simulink library "base_lib"  (R2023a)
settings: Solver=VariableStepAuto  StartTime=0.0  StopTime=10.0  RelTol=1e-3
(part 4 of 4)

== matlab function base_lib/F0021_R1234yf/F0021_dudrho.m ==
  data: T input; du_drho output; rho input
function du_drho = R1234yf_dudrho(T,rho)
%R1234yf_dudrho
%    DU_DRHO = R1234yf_dudrho(T,RHO)

%    This function was generated by the Symbolic Math Toolbox version 9.3.
%    19-Oct-2023 14:13:06

t2 = rho.^2;
t3 = rho.^3;
t4 = 1.0./T;
t7 = rho./4.17e+3;
t12 = rho.*1.863257595362559e-6;
t15 = rho.*1.173162189672722e-7;
t19 = rho.*6.716928615381076e-7;
t20 = rho.*1.53661243666937e-7;
t21 = rho.*1.213417755004629e-7;
t5 = t4.^2;
t6 = t4.^3;
t8 = -t7;
t9 = t4.*5.8856e+4;
t11 = t4.*3.6785e+2;
t13 = t4.*7.94556e+4;
t14 = t2./1.73889e+7;
t16 = t4.*1.044694e+3;
t17 = t7-4.1e+1./2.5e+1;
t27 = t4.*6.54773e+2;
t28 = t4.*1.699467e+3;
t29 = t7-9.1e+1./1.0e+2;
t30 = t7-8.9e+1./1.25e+2;
t31 = t7-3.59e+2./5.0e+2;
t39 = t7-6.77e+2./1.0e+3;
t60 = t12-1.274244604316547e-2;
t68 = t15-3.483165467625899e-4;
t79 = t19-2.011088729016787e-3;
t81 = t20-5.830983213429257e-4;
t82 = t21-3.425587529976019e-4;
t10 = exp(t8);
t18 = -t14;
t22 = t11.^(2.0./5.0);
t23 = t11.^(5.0./2.0);
t24 = t11.^(7.0./2.0);
t25 = t11.^(7.0./5.0);
t32 = t11-6.0./5.0;
t33 = t11.^(1.0./2.0e+1);
t34 = t17.^2;
t35 = t11.^(1.9e+1./2.5e+1);
t36 = t11.^(3.2e+1./2.5e+1);
t37 = t11.^(3.6e+1./2.5e+1);
t38 = t9-2.048e+2;
t40 = t11-3.2e+1./2.5e+1;
t41 = t11-2.3e+1./5.0e+1;
t42 = 1.0./t11.^(3.0./1.0e+2);
t43 = t29.^2;
t44 = t30.^2;
t45 = t31.^2;
t47 = t11-6.7e+1./1.0e+2;
t48 = t11-1.13e+2./1.0e+2;
t49 = t13-2.592e+2;
t50 = t39.^2;
t63 = t16-3.2092;
t69 = t27-8.188e-1;
t72 = t28-3.0954;
t26 = exp(t18);
t46 = t32.^2;
t51 = t40.^2;
t52 = t41.^2;
t54 = t47.^2;
t55 = t48.^2;
t56 = t34.*(8.1e+1./5.0);
t61 = t44.*(5.1e+1./5.0e+1);
t65 = t45.*(1.46e+2./2.5e+1);
t66 = t43.*(1.67e+2./1.25e+2);
t73 = t50.*(2.11e+2./2.0e+2);
t53 = t46.*1.08e+2;
t58 = -t56;
t59 = t51.*8.0e+1;
t64 = -t61;
t67 = -t65;
t70 = -t66;
t71 = t52.*(8.9e+1./1.0e+2);
t75 = t55.*(7.1e+1./5.0e+1);
t76 = -t73;
t78 = t54.*(2.31e+2./1.0e+2);
t57 = -t53;
t62 = -t59;
t74 = -t71;
t77 = -t75;
t80 = -t78;
t83 = t57+t58;
t85 = t62+t67;
t87 = t64+t77;
t89 = t70+t80;
t90 = t74+t76;
t84 = exp(t83);
t86 = exp(t85);
t88 = exp(t87);
t91 = exp(t89);
t92 = exp(t90);
et1 = t3.*1.858131002604336e-12-t26.*t36.*2.023446617579852;
et2 = t2.*t86.*(-1.452200134424495e-7)-t5.*t91.*1.422328005554134e+5;
et3 = t22.*t88.*1.427255066297698-rho.*t42.^2.*1.59640689065627e-4;
et4 = t2.*1.0./t11.^(3.1e+1./5.0e+1).*8.453302832006239e-9+1.0./t11.^(1.7e+1./2.5e+1).*3.630762837322852e-1;
et5 = 1.0./t11.^(7.1e+1./1.0e+3).*(-1.60479554422836)+rho.^7.*t10.*t33.*9.468704878352454e-28;
et6 = t2.^3.*t10.*t33.*(-2.763914953991081e-23)+t2.^2.*t26.*t35.*5.274136083584932e-15;
et7 = rho.*t10.*t42.*2.322094583878085e-4-rho.*t26.*t37.*5.981304050145462e-4;
et8 = rho.*t23.*t84.*4.221246493387974e-7-t2.*t10.*t42.*2.784286071796265e-8;
et9 = t2.*t26.*t35.*(-1.37567137415775e-7)+t2.*t26.*t36.*2.327285357417493e-7;
et10 = t3.*t26.*t37.*3.439725370866163e-11-t2.*t23.*t92.*8.74770499448078e-8;
et11 = t3.*t79.*t86.*4.840667114748315e-8+t6.*t72.*t91.*1.74401118947696e+7;
et12 = t25.*t63.*t88.*(-1.019467904498356)-rho.*t24.*t49.*t84.*1.206070426682278e-7;
et13 = rho.*t5.*t81.*t91.*1.422328005554134e+5-rho.*t22.*t68.*t88.*1.427255066297698;
et14 = t2.*t4.*t38.*t86.*5.341918194480503e-5-t2.*t23.*t60.*t84.*2.110623246693987e-7;
et15 = t2.*t24.*t69.*t92.*2.499344284137366e-8+t3.*t23.*t82.*t92.*2.915901664826927e-8;
et16 = rho.*t25.*t63.*t68.*t88.*1.019467904498356-rho.*t6.*t72.*t81.*t91.*1.74401118947696e+7;
et17 = t3.*t4.*t38.*t79.*t86.*(-1.780639398160168e-5)+t2.*t24.*t49.*t60.*t84.*6.030352133411391e-8;
et18 = t3.*t24.*t69.*t82.*t92.*(-8.331147613791219e-9);
du_drho = et1+et2+et3+et4+et5+et6+et7+et8+et9+et10+et11+et12+et13+et14+et15+et16+et17+et18;
end

== matlab function base_lib/F0021_R1234yf/F0021_dvapsat.m ==
  data: T input; dvap output
function dvap = F0021_dvapsat(T)

% critical Temp & density
Tc   =     367.85; % [K]
% rhoc =     4170.0; % [mol/m3]

T = min(T, Tc);
T = max(T, 0);

% coefficients
x = [ 8.5116; -7.9050; 1.6189; 2.6394; -1.3847 ];

% saturated vapor density
Tr   = T ./ Tc;
th   = 1 ./ (1 - Tr);
A    = [ ones(size(Tr)), log(th).^(-1.5), log(th).^(-2), log(th).^(-3), log(th).^(-4) ];
dvap = exp(A*x);


end

== matlab function base_lib/F0021_R1234yf/F0021_g.m ==
  data: T input; g output; rho input
function g = F0021_g(T,rho)
%R1234yf_g
%    G = R1234yf_g(T,RHO)

%    This function was generated by the Symbolic Math Toolbox version 9.3.
%    16-Oct-2023 15:47:52

t2 = rho.^2;
t3 = rho.^3;
t5 = rho.^7;
t6 = 1.0./T;
t8 = rho./4.17e+3;
t4 = t2.^2;
t7 = t6.^3;
t9 = -t8;
t11 = t6.*3.6785e+2;
t12 = t2./1.73889e+7;
t13 = t8-4.1e+1./2.5e+1;
t18 = t8-9.1e+1./1.0e+2;
t19 = t8-8.9e+1./1.25e+2;
t20 = t8-3.59e+2./5.0e+2;
t30 = t8-6.77e+2./1.0e+3;
t10 = exp(t9);
t14 = -t12;
t15 = t11.^(7.0./2.0);
t16 = t11.^(7.0./5.0);
t21 = t11-6.0./5.0;
t22 = t13.^2;
t23 = t11.^(8.0./2.5e+1);
t24 = t11.^(2.1e+1./2.0e+1);
t25 = t11.^(1.9e+1./5.0e+1);
t26 = t11.^(4.4e+1./2.5e+1);
t28 = t11.^(6.1e+1./2.5e+1);
t29 = t11.^(4.7e+1./5.0e+1);
t31 = t11-3.2e+1./2.5e+1;
t32 = t11-2.3e+1./5.0e+1;
t33 = t18.^2;
t34 = t19.^2;
t35 = t20.^2;
t37 = t11.^(9.7e+1./1.0e+2);
t38 = t11-6.7e+1./1.0e+2;
t39 = t11-1.13e+2./1.0e+2;
t40 = t30.^2;
t43 = t11.^(9.29e+2./1.0e+3);
t17 = exp(t14);
t27 = t25.^6;
t36 = t21.^2;
t41 = t31.^2;
t42 = t32.^2;
t45 = t38.^2;
t46 = t39.^2;
t47 = t22.*(8.1e+1./5.0);
t51 = t34.*(5.1e+1./5.0e+1);
t54 = t35.*(1.46e+2./2.5e+1);
t55 = t33.*(1.67e+2./1.25e+2);
t59 = t40.*(2.11e+2./2.0e+2);
t76 = t2.*t10.*t37.*3.913566700596357e-8;
t77 = t5.*t10.*t24.*1.229509534838242e-27;
t44 = t36.*1.08e+2;
t49 = -t47;
t50 = t41.*8.0e+1;
t53 = -t51;
t56 = -t54;
t57 = -t55;
t58 = t42.*(8.9e+1./1.0e+2);
t61 = t46.*(7.1e+1./5.0e+1);
t62 = -t59;
t64 = t45.*(2.31e+2./1.0e+2);
t48 = -t44;
t52 = -t50;
t60 = -t58;
t63 = -t61;
t65 = -t64;
t66 = t48+t49;
t68 = t52+t56;
t70 = t53+t63;
t72 = t57+t65;
t73 = t60+t62;
t67 = exp(t66);
t69 = exp(t68);
t71 = exp(t70);
t74 = exp(t72);
t75 = exp(t73);
et1 = t23.*1.546958-t43.*2.355237-t76+t77-rho.*t29.*2.315508393285372e-4+t3.*t6.*9.319180196722149e-10;
et2 = t2.*t25.*3.033007263254145e-8-t17.*t27.*1.210006-t7.*t74.*2.377824987227386e+7+t16.*t71.*1.389966;
et3 = t2.^3.*t10.*t24.*(-3.588938332192827e-23)-rho.*t17.*t28.*3.342232613908873e-4+rho.*t10.*t37.*3.263914628297362e-4+rho.*t15.*t67.*1.644384172661871e-7;
et4 = t2.*t17.*t26.*(-1.06569432224005e-7)+t2.*t17.*t27.*1.391699302428561e-7+t4.*t17.*t26.*4.085726420264459e-15+t3.*t17.*t28.*1.922049476337705e-11;
et5 = t2.*t6.*t69.*(-7.283294189396684e-5)-t2.*t15.*t75.*3.407663509480186e-8-rho.*t16.*t71.*(rho.*4.892086330935252e-4-1.45248).*3.333251798561151e-4;
et6 = rho.*t7.*t74.*(rho.*6.407673860911271e-4-2.43152).*5.702218194789895e+3-t2.*t15.*t67.*(rho.*7.769784172661871e-3-5.3136e+1).*1.971683660266032e-11;
et7 = t3.*t6.*t69.*(rho.*2.800959232613909e-3-8.38624).*5.821977769301905e-9+t3.*t15.*t75.*(rho.*5.059952038369305e-4-1.42847).*2.723951646267135e-12;
et8 = t6.*2.95847224925e+3+t76-t77+log(-exp(t6.*-7.18e+2)+1.0).*7.549+log(-exp(t6.*-8.77e+2)+1.0).*1.537+log(-exp(t6.*-1.755e+3)+1.0).*7.455+log(-exp(t6.*-4.465e+3)+1.0).*(2.03e+2./1.0e+2)+log(t8)+log(t11).*(6.18e+2./1.25e+2)+rho.*t23.*3.709731414868106e-4;
et9 = rho.*t43.*(-5.64805035971223e-4)+t4.*t6.*5.587038487243495e-14+t3.*t25.*2.424466237613225e-12-t2.*t29.*2.776388960773827e-8+t8.*(et1+et2+et3+et4+et5+et6+et7);
et10 = rho.*t17.*t27.*(-2.901693045563549e-4)-rho.*t7.*t74.*5.702218194789895e+3+rho.*t16.*t71.*3.333251798561151e-4-t3.*t17.*t26.*8.518739586251397e-12;
et11 = t2.*t17.*t28.*(-4.007473158164116e-8)-t3.*t6.*t69.*5.821977769301905e-9+t2.*t15.*t67.*1.971683660266032e-11-t3.*t15.*t75.*2.723951646267135e-12;
et12 = -1.1837928e+1;
g = T.*(et8+et9+et10+et11+et12).*8.314472;
end

== matlab function base_lib/F0021_R1234yf/F0021_h.m ==
  data: T input; h output; rho input
function h = F0021_h(T,rho)
%R1234yf_h
%    H = R1234yf_h(T,RHO)

%    This function was generated by the Symbolic Math Toolbox version 9.3.
%    16-Oct-2023 15:47:51

t2 = rho.^2;
t3 = rho.^3;
t5 = rho.^7;
t6 = 1.0./T;
t8 = rho./4.17e+3;
t4 = t2.^2;
t7 = t6.^3;
t9 = t6.*7.18e+2;
t10 = t6.*8.77e+2;
t11 = t6.*1.755e+3;
t12 = t6.*4.465e+3;
t13 = -t8;
t23 = t6.*3.6785e+2;
t24 = t2./1.73889e+7;
t25 = t8-4.1e+1./2.5e+1;
t31 = t8-9.1e+1./1.0e+2;
t32 = t8-8.9e+1./1.25e+2;
t33 = t8-3.59e+2./5.0e+2;
t40 = t8-6.77e+2./1.0e+3;
t14 = -t9;
t15 = -t10;
t16 = -t11;
t17 = -t12;
t18 = exp(t13);
t26 = -t24;
t27 = t23.^(5.0./2.0);
t28 = t23.^(7.0./2.0);
t29 = t23.^(7.0./5.0);
t34 = t23-6.0./5.0;
t35 = t25.^2;
t36 = t23.^(2.1e+1./2.0e+1);
t37 = t23.^(4.4e+1./2.5e+1);
t38 = t23.^(5.7e+1./2.5e+1);
t39 = t23.^(6.1e+1./2.5e+1);
t41 = t23-3.2e+1./2.5e+1;
t42 = t23-2.3e+1./5.0e+1;
t43 = t31.^2;
t44 = t32.^2;
t45 = t33.^2;
t47 = t23.^(9.7e+1./1.0e+2);
t48 = t23-6.7e+1./1.0e+2;
t49 = t23-1.13e+2./1.0e+2;
t50 = t40.^2;
t19 = exp(t14);
t20 = exp(t15);
t21 = exp(t16);
t22 = exp(t17);
t30 = exp(t26);
t46 = t34.^2;
t51 = t41.^2;
t52 = t42.^2;
t54 = t48.^2;
t55 = t49.^2;
t56 = t35.*(8.1e+1./5.0);
t60 = t44.*(5.1e+1./5.0e+1);
t63 = t45.*(1.46e+2./2.5e+1);
t64 = t43.*(1.67e+2./1.25e+2);
t68 = t50.*(2.11e+2./2.0e+2);
t53 = t46.*1.08e+2;
t58 = -t56;
t59 = t51.*8.0e+1;
t62 = -t60;
t65 = -t63;
t66 = -t64;
t67 = t52.*(8.9e+1./1.0e+2);
t70 = t55.*(7.1e+1./5.0e+1);
t71 = -t68;
t73 = t54.*(2.31e+2./1.0e+2);
t57 = -t53;
t61 = -t59;
t69 = -t67;
t72 = -t70;
t74 = -t73;
t75 = t57+t58;
t77 = t61+t65;
t79 = t62+t72;
t81 = t66+t74;
t82 = t69+t71;
t76 = exp(t75);
t78 = exp(t77);
t80 = exp(t79);
t83 = exp(t81);
t84 = exp(t82);
et1 = T.*(-1.344026097594128e-2)-t4.*1.518836071019028e-16+(t19.*1.473476145167867e+1)./(t19-1.0)+(t20.*3.66439853201033)./(t20-1.0)+(t21.*3.556755470980019e+1)./(t21-1.0)+(t22.*2.464034253092293e+1)./(t22-1.0)+t3.*t78.*1.582704300476255e-11;
et2 = rho.*1.0./t23.^(1.7e+1./2.5e+1).*(-1.187114052757794e-4)+rho.*1.0./t23.^(7.1e+1./1.0e+3).*5.247038784172661e-4+t2.*1.0./t23.^(3.0./5.0e+1).*2.609805623127397e-8;
et3 = t3.*1.0./t23.^(3.1e+1./5.0e+1).*(-9.212971702930256e-13)+rho.*t6.^2.*t83.*4.650443002411223e+1-rho.*t23.^(2.0./5.0).*t80.*4.666552517985612e-4;
et4 = rho.*t23.^(3.2e+1./2.5e+1).*t30.*6.615860143884892e-4+t5.*t18.*t23.^(1.0./2.0e+1).*1.290985011580154e-27+t3.*t23.^(1.9e+1./2.5e+1).*t30.*1.499298167180246e-11;
et5 = t2.*t23.^(3.6e+1./2.5e+1).*t30.*9.778234505920443e-8-t2.*t18.*1.0./t23.^(3.0./1.0e+2).*3.796159699578467e-8-t2.*t27.*t76.*6.900892810931111e-11;
et6 = t3.*t27.*t84.*9.533830761934972e-12+rho.*t29.*t80.*(t6.*1.044694e+3-3.2092).*3.333251798561151e-4-rho.*t7.*t83.*(t6.*1.699467e+3-3.0954).*5.702218194789895e+3;
et7 = t3.*t6.*t78.*(t6.*5.8856e+4-2.048e+2).*(-5.821977769301905e-9)+t2.*t28.*t76.*(t6.*7.94556e+4-2.592e+2).*1.971683660266032e-11;
et8 = t3.*t28.*t84.*(t6.*6.54773e+2-8.188e-1).*(-2.723951646267135e-12)-8.042605;
et9 = t3.*t6.*9.319180196722149e-10-t30.*t38.*1.210006-t7.*t83.*2.377824987227386e+7+t29.*t80.*1.389966;
et10 = rho.*t23.^(4.7e+1./5.0e+1).*(-2.315508393285372e-4)+t2.*t23.^(1.9e+1./5.0e+1).*3.033007263254145e-8+t23.^(8.0./2.5e+1).*1.546958-t23.^(9.29e+2./1.0e+3).*2.355237;
et11 = t2.^3.*t18.*t36.*(-3.588938332192827e-23)+rho.*t18.*t47.*3.263914628297362e-4-rho.*t30.*t39.*3.342232613908873e-4+rho.*t28.*t76.*1.644384172661871e-7;
et12 = t5.*t18.*t36.*1.229509534838242e-27-t2.*t18.*t47.*3.913566700596357e-8-t2.*t30.*t37.*1.06569432224005e-7+t2.*t30.*t38.*1.391699302428561e-7;
et13 = t4.*t30.*t37.*4.085726420264459e-15+t3.*t30.*t39.*1.922049476337705e-11-t2.*t6.*t78.*7.283294189396684e-5-t2.*t28.*t84.*3.407663509480186e-8;
et14 = rho.*t29.*t80.*(rho.*4.892086330935252e-4-1.45248).*(-3.333251798561151e-4)+rho.*t7.*t83.*(rho.*6.407673860911271e-4-2.43152).*5.702218194789895e+3;
et15 = t2.*t28.*t76.*(rho.*7.769784172661871e-3-5.3136e+1).*(-1.971683660266032e-11)+t3.*t6.*t78.*(rho.*2.800959232613909e-3-8.38624).*5.821977769301905e-9;
et16 = t3.*t28.*t84.*(rho.*5.059952038369305e-4-1.42847).*2.723951646267135e-12;
h = T.*(t6.*(et1+et2+et3+et4+et5+et6+et7+et8).*(-3.6785e+2)+t8.*(et9+et10+et11+et12+et13+et14+et15+et16)+1.0).*8.314472;
end

== matlab function base_lib/F0021_R1234yf/F0021_p.m ==
  data: T input; p output; rho input
function p = F0021_p(T,rho)
%R1234yf_p
%    P = R1234yf_p(T,RHO)

%    This function was generated by the Symbolic Math Toolbox version 9.3.
%    16-Oct-2023 15:47:49

t2 = rho.^2;
t3 = rho.^3;
t4 = 1.0./T;
t6 = rho./4.17e+3;
t5 = t4.^3;
t7 = -t6;
t9 = t4.*3.6785e+2;
t10 = t2./1.73889e+7;
t11 = t6-4.1e+1./2.5e+1;
t16 = t6-9.1e+1./1.0e+2;
t17 = t6-8.9e+1./1.25e+2;
t18 = t6-3.59e+2./5.0e+2;
t25 = t6-6.77e+2./1.0e+3;
t8 = exp(t7);
t12 = -t10;
t13 = t9.^(7.0./2.0);
t14 = t9.^(7.0./5.0);
t19 = t9-6.0./5.0;
t20 = t11.^2;
t21 = t9.^(2.1e+1./2.0e+1);
t22 = t9.^(4.4e+1./2.5e+1);
t23 = t9.^(5.7e+1./2.5e+1);
t24 = t9.^(6.1e+1./2.5e+1);
t26 = t9-3.2e+1./2.5e+1;
t27 = t9-2.3e+1./5.0e+1;
t28 = t16.^2;
t29 = t17.^2;
t30 = t18.^2;
t32 = t9.^(9.7e+1./1.0e+2);
t33 = t9-6.7e+1./1.0e+2;
t34 = t9-1.13e+2./1.0e+2;
t35 = t25.^2;
t15 = exp(t12);
t31 = t19.^2;
t36 = t26.^2;
t37 = t27.^2;
t39 = t33.^2;
t40 = t34.^2;
t41 = t20.*(8.1e+1./5.0);
t45 = t29.*(5.1e+1./5.0e+1);
t48 = t30.*(1.46e+2./2.5e+1);
t49 = t28.*(1.67e+2./1.25e+2);
t53 = t35.*(2.11e+2./2.0e+2);
t38 = t31.*1.08e+2;
t43 = -t41;
t44 = t36.*8.0e+1;
t47 = -t45;
t50 = -t48;
t51 = -t49;
t52 = t37.*(8.9e+1./1.0e+2);
t55 = t40.*(7.1e+1./5.0e+1);
t56 = -t53;
t58 = t39.*(2.31e+2./1.0e+2);
t42 = -t38;
t46 = -t44;
t54 = -t52;
t57 = -t55;
t59 = -t58;
t60 = t42+t43;
t62 = t46+t50;
t64 = t47+t57;
t66 = t51+t59;
t67 = t54+t56;
t61 = exp(t60);
t63 = exp(t62);
t65 = exp(t64);
t68 = exp(t66);
t69 = exp(t67);
et1 = t3.*t4.*9.319180196722149e-10-t15.*t23.*1.210006-t5.*t68.*2.377824987227386e+7+t14.*t65.*1.389966;
et2 = rho.*t9.^(4.7e+1./5.0e+1).*(-2.315508393285372e-4)+t2.*t9.^(1.9e+1./5.0e+1).*3.033007263254145e-8+t9.^(8.0./2.5e+1).*1.546958-t9.^(9.29e+2./1.0e+3).*2.355237;
et3 = rho.^7.*t8.*t21.*1.229509534838242e-27-t2.^3.*t8.*t21.*3.588938332192827e-23+t2.^2.*t15.*t22.*4.085726420264459e-15;
et4 = rho.*t15.*t24.*(-3.342232613908873e-4)+rho.*t8.*t32.*3.263914628297362e-4+rho.*t13.*t61.*1.644384172661871e-7-t2.*t15.*t22.*1.06569432224005e-7;
et5 = t2.*t15.*t23.*1.391699302428561e-7-t2.*t8.*t32.*3.913566700596357e-8+t3.*t15.*t24.*1.922049476337705e-11-t2.*t4.*t63.*7.283294189396684e-5;
et6 = t2.*t13.*t69.*(-3.407663509480186e-8)-rho.*t14.*t65.*(rho.*4.892086330935252e-4-1.45248).*3.333251798561151e-4+rho.*t5.*t68.*(rho.*6.407673860911271e-4-2.43152).*5.702218194789895e+3;
et7 = t2.*t13.*t61.*(rho.*7.769784172661871e-3-5.3136e+1).*(-1.971683660266032e-11)+t3.*t4.*t63.*(rho.*2.800959232613909e-3-8.38624).*5.821977769301905e-9;
et8 = t3.*t13.*t69.*(rho.*5.059952038369305e-4-1.42847).*2.723951646267135e-12;
p = T.*rho.*(t6.*(et1+et2+et3+et4+et5+et6+et7+et8)+1.0).*8.314472;
end

== matlab function base_lib/F0003_pukrushpan2004/F0003_reactionFlow.m ==
  data: I input; W_an output; W_ca output
function [W_an, W_ca] = F0003_reactionFlow(I)
% constants
F     = 96485; % [C/mol]  - Faradays constant
M_H2  = 0.002; % [kg/mol] - hydrogen molecular weight
M_O2  = 0.032; % [kg/mol] - oxygen   molecular weight
% M_N2  = 0.028; % [kg/mol] - nitrogen molecular weight
M_H2O = 0.018; % [kg/mol] - water    molecular weight

% reaction flows
W_H2_rct  = I * M_H2  /(2*F);
W_O2_rct  = I * M_O2  /(4*F);
W_H2O_rct = I * M_H2O /(2*F);

% output
W_an = [-W_H2_rct;         0;         0; 0];
W_ca = [        0; -W_O2_rct; W_H2O_rct; 0]; 
end

== matlab function base_lib/F0021_R1234yf/F0021_psat.m ==
  data: T input; p_sat output
function p_sat = F0021_psat(T)
% Van Laar, J. L Res Tray Chim 39 (1920) 21
% fit to data from 
% Richter, Mclinden, Lemmon Journal of. Chem. E (2011)

% critical Temp & density
Tc   =     367.85; % [K]

T = max(T,0);
T = min(T, Tc);


% R1234yf coefficients
n = [ -4.893666065312787; 
       0.111013414194105; 
       0.000025221844863;
       -0.015565681357114] * 1e3;

% saturation pressure
p_sat = exp( n(1) .* (1./T) + n(2) + n(3) .* T + n(4) .* log(T) ); 
end

== matlab function base_lib/F0021_R1234yf/F0021_s.m ==
  data: T input; s output; rho input
function s = F0021_s(T,rho)
%R1234yf_s
%    S = R1234yf_s(T,RHO)

%    This function was generated by the Symbolic Math Toolbox version 9.3.
%    16-Oct-2023 15:47:49

t2 = rho.^2;
t3 = rho.^3;
t5 = rho.^7;
t6 = 1.0./T;
t8 = rho./4.17e+3;
t4 = t2.^2;
t7 = t6.^3;
t9 = t6.*7.18e+2;
t10 = t6.*8.77e+2;
t11 = t6.*1.755e+3;
t12 = t6.*4.465e+3;
t13 = -t8;
t23 = t6.*3.6785e+2;
t24 = t2./1.73889e+7;
t25 = t8-4.1e+1./2.5e+1;
t31 = t8-9.1e+1./1.0e+2;
t32 = t8-8.9e+1./1.25e+2;
t33 = t8-3.59e+2./5.0e+2;
t36 = t8-6.77e+2./1.0e+3;
t14 = -t9;
t15 = -t10;
t16 = -t11;
t17 = -t12;
t18 = exp(t13);
t26 = -t24;
t27 = t23.^(5.0./2.0);
t28 = t23.^(7.0./2.0);
t29 = t23.^(7.0./5.0);
t34 = t23-6.0./5.0;
t35 = t25.^2;
t37 = t23-3.2e+1./2.5e+1;
t38 = t23-2.3e+1./5.0e+1;
t39 = t31.^2;
t40 = t32.^2;
t41 = t33.^2;
t43 = t23-6.7e+1./1.0e+2;
t44 = t23-1.13e+2./1.0e+2;
t45 = t36.^2;
t19 = exp(t14);
t20 = exp(t15);
t21 = exp(t16);
t22 = exp(t17);
t30 = exp(t26);
t42 = t34.^2;
t46 = t37.^2;
t47 = t38.^2;
t49 = t43.^2;
t50 = t44.^2;
t51 = t35.*(8.1e+1./5.0);
t55 = t40.*(5.1e+1./5.0e+1);
t58 = t41.*(1.46e+2./2.5e+1);
t59 = t39.*(1.67e+2./1.25e+2);
t63 = t45.*(2.11e+2./2.0e+2);
t48 = t42.*1.08e+2;
t53 = -t51;
t54 = t46.*8.0e+1;
t57 = -t55;
t60 = -t58;
t61 = -t59;
t62 = t47.*(8.9e+1./1.0e+2);
t65 = t50.*(7.1e+1./5.0e+1);
t66 = -t63;
t68 = t49.*(2.31e+2./1.0e+2);
t52 = -t48;
t56 = -t54;
t64 = -t62;
t67 = -t65;
t69 = -t68;
t70 = t52+t53;
t72 = t56+t60;
t74 = t57+t67;
t76 = t61+t69;
t77 = t64+t66;
t71 = exp(t70);
t73 = exp(t72);
t75 = exp(t74);
t78 = exp(t76);
t79 = exp(t77);
et1 = T.*(-1.344026097594128e-2)-t4.*1.518836071019028e-16+(t19.*1.473476145167867e+1)./(t19-1.0)+(t20.*3.66439853201033)./(t20-1.0)+(t21.*3.556755470980019e+1)./(t21-1.0)+(t22.*2.464034253092293e+1)./(t22-1.0)+t3.*t73.*1.582704300476255e-11;
et2 = rho.*1.0./t23.^(1.7e+1./2.5e+1).*(-1.187114052757794e-4)+rho.*1.0./t23.^(7.1e+1./1.0e+3).*5.247038784172661e-4+t2.*1.0./t23.^(3.0./5.0e+1).*2.609805623127397e-8;
et3 = t3.*1.0./t23.^(3.1e+1./5.0e+1).*(-9.212971702930256e-13)+rho.*t6.^2.*t78.*4.650443002411223e+1-rho.*t23.^(2.0./5.0).*t75.*4.666552517985612e-4;
et4 = rho.*t23.^(3.2e+1./2.5e+1).*t30.*6.615860143884892e-4+t5.*t18.*t23.^(1.0./2.0e+1).*1.290985011580154e-27+t3.*t23.^(1.9e+1./2.5e+1).*t30.*1.499298167180246e-11;
et5 = t2.*t23.^(3.6e+1./2.5e+1).*t30.*9.778234505920443e-8-t2.*t18.*1.0./t23.^(3.0./1.0e+2).*3.796159699578467e-8-t2.*t27.*t71.*6.900892810931111e-11;
et6 = t3.*t27.*t79.*9.533830761934972e-12+rho.*t29.*t75.*(t6.*1.044694e+3-3.2092).*3.333251798561151e-4-rho.*t7.*t78.*(t6.*1.699467e+3-3.0954).*5.702218194789895e+3;
et7 = t3.*t6.*t73.*(t6.*5.8856e+4-2.048e+2).*(-5.821977769301905e-9)+t2.*t28.*t71.*(t6.*7.94556e+4-2.592e+2).*1.971683660266032e-11;
et8 = t3.*t28.*t79.*(t6.*6.54773e+2-8.188e-1).*(-2.723951646267135e-12)-8.042605;
et9 = t6.*(-2.459813467916615e+4)-log(-t19+1.0).*6.2765949128e+1-log(-t20+1.0).*1.2779343464e+1;
et10 = log(-t21+1.0).*(-6.198438876e+1)-log(-t22+1.0).*1.687837816e+1-log(t8).*8.314472-log(t23).*4.1106749568e+1;
et11 = t4.*t6.*(-4.64532750651084e-13)-t6.*(et1+et2+et3+et4+et5+et6+et7+et8).*3.0584785252e+3;
et12 = rho.*t23.^(8.0./2.5e+1).*(-3.084445797644125e-3)+rho.*t23.^(9.29e+2./1.0e+3).*4.696055657041726e-3;
et13 = t3.*t23.^(1.9e+1./5.0e+1).*(-2.015815664758051e-11)+t2.*t23.^(4.7e+1./5.0e+1).*2.308420827546308e-7;
et14 = rho.*t23.^(5.7e+1./2.5e+1).*t30.*2.412604557993285e-3+t5.*t18.*t23.^(2.1e+1./2.0e+1).*1.022272260114558e-26;
et15 = t3.*t23.^(4.4e+1./2.5e+1).*t30.*7.082882176517883e-11+t2.*t23.^(6.1e+1./2.5e+1).*t30.*3.332002336430711e-7;
et16 = t2.*t18.*t23.^(9.7e+1./1.0e+2).*(-3.25392407522408e-7)+rho.*t7.*t78.*4.741093351847113e+4;
et17 = rho.*t29.*t75.*(-2.771422874808633e-3)+t3.*t6.*t73.*4.840667114748315e-8;
et18 = t2.*t28.*t71.*(-1.639350858613943e-10)+t3.*t28.*t79.*2.2648219692242e-11;
et19 = 1.06740592894016e+2;
s = et9+et10+et11+et12+et13+et14+et15+et16+et17+et18+et19;
end

== matlab function base_lib/F0022_heatPump/F0022_LockhartMartinelliParameter.m ==
  data: x input; X_tt output; rho_g input; rho_f input; mu_g input; mu_f input
function X_tt = F0022_LockhartMartinelliParameter(x, rho_g, rho_f, mu_g, mu_f)

% Lockhart-Martinelly Parameter (nuclear-power.com)
X_tt = ((1-x)./x).^0.9 .* (rho_g ./ rho_f).^0.5 .* (mu_f ./ mu_g ).^0.1;


end

== matlab function base_lib/F0022_heatPump/F0022_OSFPHEX.m ==
  data: G input; h output; x input; rho_f input; rho_g input; cp_f input; cp_g input; mu_f input; mu_g input; k_f input; k_g input; sigma input; par parameter
function h = F0022_OSFPHEX(G, x, rho_f, rho_g, cp_f, cp_g, mu_f, mu_g, k_f, k_g, sigma, par)

% parameters
D_h = par.D_h;

% output size
h = zeros(size(x));

% Bond number
g   = 9.81;
B_d = g .* (rho_f - rho_g) .* D_h.^2 ./ sigma;

% liquid & gas Prandtl number
Pr_f = cp_f .* mu_f ./ k_f;
Pr_g = cp_g .* mu_g ./ k_g;

% minimum mass flux
G = max(G, 1);

% refrigerant side heat transfer coefficient
G_eq  = G .* ( (1-x) + (rho_f./rho_g).^0.5 .* x );
Re_f  = G    .* D_h ./ mu_f;
Re_g  = G    .* D_h ./ mu_g;
Re_eq = G_eq .* D_h ./ mu_f;
Nu    = 3.918 .* Re_eq.^0.505 .* Re_f.^(-0.1354) .* B_d.^0.213 .* Pr_f.^(1/3);
h_tp     = Nu .* k_f ./ D_h;

% single phase correlation
h_f = 0.494 .* G .* cp_f .* Re_f.^(-0.426) .* Pr_f.^(-2/3);
h_g = 0.494 .* G .* cp_g .* Re_g.^(-0.426) .* Pr_g.^(-2/3);

% smooth transition to subcooled liquid & superheated vapor
y = (x-0.1) / 0.1;
y = tanh(y*5)/2 + 1/2;
z =  (x-0.90) / 0.1;
z = tanh(z*5)/2 + 1/2;

h = h_tp .* y .* (1-z) + h_f .* (1-y) + h_g .* z;

% output
% h       = h_tp;
% h(x==0) = h_f(x==0);
% h(x==1) = h_g(x==1);



end

== matlab function base_lib/F0022_heatPump/F0022_artificialMass.m ==
  data: p input; m output; par parameter
function m = F0022_artificialMass(p, par)

% parameters
B       = par.BV .* par.V;
rho_ref = par.rho_ref;
V       = par.V;

% artificial mass
m = V .* rho_ref .* (p./B + 1);


end

== matlab function base_lib/F0022_heatPump/F0022_artificialPressure.m ==
  data: m input; p output; par parameter
function p = F0022_artificialPressure(m, par)

% parameters
V = par.V;
B = par.BV .* par.V;
rho_ref = par.rho_ref;


% artificial pressure
p = B .* (m./(V .* rho_ref) - 1); 

end

== matlab function base_lib/F0021_R1234yf/F0021_u.m ==
  data: T input; u output; rho input
function u = F0021_u(T,rho)
%R1234yf_u
%    U = R1234yf_u(T,RHO)

%    This function was generated by the Symbolic Math Toolbox version 9.3.
%    16-Oct-2023 15:47:50

t2 = rho.^2;
t3 = rho.^3;
t4 = 1.0./T;
t5 = rho./4.17e+3;
t6 = t4.*7.18e+2;
t7 = t4.*8.77e+2;
t8 = t4.*1.755e+3;
t9 = t4.*4.465e+3;
t10 = -t5;
t20 = t4.*3.6785e+2;
t21 = t2./1.73889e+7;
t22 = t5-4.1e+1./2.5e+1;
t27 = t5-9.1e+1./1.0e+2;
t28 = t5-8.9e+1./1.25e+2;
t29 = t5-3.59e+2./5.0e+2;
t32 = t5-6.77e+2./1.0e+3;
t11 = -t6;
t12 = -t7;
t13 = -t8;
t14 = -t9;
t15 = exp(t10);
t23 = -t21;
t24 = t20.^(5.0./2.0);
t25 = t20.^(7.0./2.0);
t30 = t20-6.0./5.0;
t31 = t22.^2;
t33 = t20-3.2e+1./2.5e+1;
t34 = t20-2.3e+1./5.0e+1;
t35 = t27.^2;
t36 = t28.^2;
t37 = t29.^2;
t39 = t20-6.7e+1./1.0e+2;
t40 = t20-1.13e+2./1.0e+2;
t41 = t32.^2;
t16 = exp(t11);
t17 = exp(t12);
t18 = exp(t13);
t19 = exp(t14);
t26 = exp(t23);
t38 = t30.^2;
t42 = t33.^2;
t43 = t34.^2;
t45 = t39.^2;
t46 = t40.^2;
t47 = t31.*(8.1e+1./5.0);
t51 = t36.*(5.1e+1./5.0e+1);
t54 = t37.*(1.46e+2./2.5e+1);
t55 = t35.*(1.67e+2./1.25e+2);
t59 = t41.*(2.11e+2./2.0e+2);
t44 = t38.*1.08e+2;
t49 = -t47;
t50 = t42.*8.0e+1;
t53 = -t51;
t56 = -t54;
t57 = -t55;
t58 = t43.*(8.9e+1./1.0e+2);
t61 = t46.*(7.1e+1./5.0e+1);
t62 = -t59;
t64 = t45.*(2.31e+2./1.0e+2);
t48 = -t44;
t52 = -t50;
t60 = -t58;
t63 = -t61;
t65 = -t64;
t66 = t48+t49;
t68 = t52+t56;
t70 = t53+t63;
t72 = t57+t65;
t73 = t60+t62;
t67 = exp(t66);
t69 = exp(t68);
t71 = exp(t70);
t74 = exp(t72);
t75 = exp(t73);
et1 = T.*4.1106749568e+1-(t16.*4.5065951473904e+4)./(t16-1.0)-(t17.*1.1207484217928e+4)./(t17-1.0)-(t18.*1.087826022738e+5)./(t18-1.0);
et2 = (t19.*(-7.53619584844e+4))./(t19-1.0)-t3.*t69.*4.840667114748315e-8;
et3 = rho.*1.0./t20.^(1.7e+1./2.5e+1).*3.630762837322852e-1-rho.*1.0./t20.^(7.1e+1./1.0e+3).*1.60479554422836;
et4 = t2.*1.0./t20.^(3.0./5.0e+1).*(-7.982034453281349e-5)+t3.*1.0./t20.^(3.1e+1./5.0e+1).*2.817767610668746e-9;
et5 = t2.^2.*4.64532750651084e-13-rho.*t4.^2.*t74.*1.422328005554134e+5;
et6 = rho.*t20.^(2.0./5.0).*t71.*1.427255066297698-rho.*t20.^(3.2e+1./2.5e+1).*t26.*2.023446617579852;
et7 = t3.*t20.^(1.9e+1./2.5e+1).*t26.*(-4.585571247192502e-8)-t2.*t20.^(3.6e+1./2.5e+1).*t26.*2.990652025072731e-4;
et8 = t2.*t15.*1.0./t20.^(3.0./1.0e+2).*1.161047291939042e-4-rho.^7.*t15.*t20.^(1.0./2.0e+1).*3.948449934272973e-24;
et9 = t2.*t24.*t67.*2.110623246693987e-7-t3.*t24.*t75.*2.915901664826927e-8;
et10 = rho.*t20.^(7.0./5.0).*t71.*(t4.*1.044694e+3-3.2092).*(-1.019467904498356);
et11 = rho.*t4.^3.*t74.*(t4.*1.699467e+3-3.0954).*1.74401118947696e+7;
et12 = t3.*t4.*t69.*(t4.*5.8856e+4-2.048e+2).*1.780639398160168e-5-t2.*t25.*t67.*(t4.*7.94556e+4-2.592e+2).*6.030352133411391e-8;
et13 = t3.*t25.*t75.*(t4.*6.54773e+2-8.188e-1).*8.331147613791219e-9+2.459813467916615e+4;
u = et1+et2+et3+et4+et5+et6+et7+et8+et9+et10+et11+et12+et13;
end

== matlab function base_lib/F0022_heatPump/F0022_compressor.m ==
  data: p_1 input; m_dot output; rho_1 input; h_1 input; p_2 input; N input; k input; P_cmp output; h_2 output; par parameter
function [m_dot, P_cmp, h_2]  = F0022_compressor(p_1, rho_1, h_1, p_2, N, k, par)
% model from Li 2013

% parameters
V_disp = par.V_disp; 
N_ref  = par.N_ref / 60;
M      = par.M;

% M = 0.1140415928; % [kg/mol]  compressor displacement
% V_disp = 0.00017; % [m3]   compressor displacement
% N_ref = 2000 / 60; % [rps]  reference speed

% suction properties
p_s   = p_1;
rho_s = rho_1 * 0.9;
h_s   = h_1;

% discharge properties
p_d = p_2;

% compressor parameters
b1    = 0.799;
b2    = -0.036;
a1    = 1.140;
a2    = 0.295;
a3    = 447.050;
Wloss = 350.000 * 2;
d1    = 1.223;
d2    = -0.206;
d3    = -0.017;
e1    = 0.507;
e2    = 0.606;
e3    = -0.113;

% reference volumetric efficieny
nv_ref = b1 + b2 .* (  (p_d./p_s ).^(1./k) );

% reference volume flow
dV_ref = nv_ref .* N_ref .* V_disp;

% reference compressor power
P_ref = p_s .* dV_ref .* a1 .* ( (p_d./p_s).^(a2 + (k-1)./k) + a3./p_d ) + Wloss; 

% volumetric efficiency ratio
nv = d1 + d2 .* (N./N_ref) + d3 .* (N./N_ref).^2;

% isentropic efficiency ratio
ni = e1 + e2 .* (N./N_ref) + e3 .* (N./N_ref).^2; 

% Compressor suction volume flow
dV_suc = dV_ref .* (N./N_ref) .* nv;
m_dot  = dV_suc  .* rho_s .* M;

% Compressor power
P_cmp = P_ref .* dV_suc ./ dV_ref .* ni;

% discharge enthalpy
h_d = M.* P_cmp ./ (m_dot + 1e-5) + h_s;
h_2 = h_d;

end

== matlab function base_lib/F0003_pukrushpan2004/F0003_vaporActivity.m ==
  data: p input; a output; P_sat input
function a = F0003_vaporActivity(p, P_sat)
a = p ./ P_sat; % [-] - water vapor activity
end

== matlab function base_lib/F0022_heatPump/F0022_coolantSideHTC.m ==
  data: G input; h output; cp input; mu input; lam input; par parameter
function h = F0022_coolantSideHTC(G, cp, mu, lam, par)

G = max(1,G);

% hydraulic diameter
D_h = par.D_h;

% Reynolds number
Re = G .* D_h ./ mu;

% Prandtl number
Pr = cp .* mu ./ lam;

% HTC
h = 0.494 .* G .* cp .* Re.^(-0.426) .* Pr.^(-2/3);

end

== matlab function base_lib/F0022_heatPump/F0022_expansionValve.m ==
  data: W input; dp output; p_us input; T_us input; rho_us input; T_sat input; alpha input; par parameter
function dp = F0022_expansionValve(W, p_us, T_us, rho_us, T_sat, alpha, par)

% parameters
M  = par.M;
Tc = par.Tc;
D  = par.D;

% constants
R = 8.314472;

% exv geometry
A = alpha .* D.^2 .* pi / 4;

% degree of subcooling
T_sub = max(T_sat - T_us, 0);

% flow coefficient
a  = [ 0.7568; -1.7428; 1.0530; 2.2342; 2.9406;  -8.4168 ];
AA = [ones(size(p_us)), alpha, alpha.^2, alpha .* T_sub/Tc, T_sub/Tc,  (T_sub/Tc).^2 ];
C  = AA * a;

% pressure drop
dp = 1./rho_us .* ( W ./ (C.*A) ).^2;

% pressure drop
% dp = p_us - p_ds;

% flow
% W = C.*A .* sqrt( rho_us .* max(dp,0) );

end
